simulink model "Lithium-ion"  (R2024b)
settings: Solver=FixedStepAuto  StartTime=0.0  StopTime=10711  FixedStep=0.001  RelTol=1e-3
(part 1 of 3)
settings Model: Creator=holthoff  LastModifiedBy=holthoff

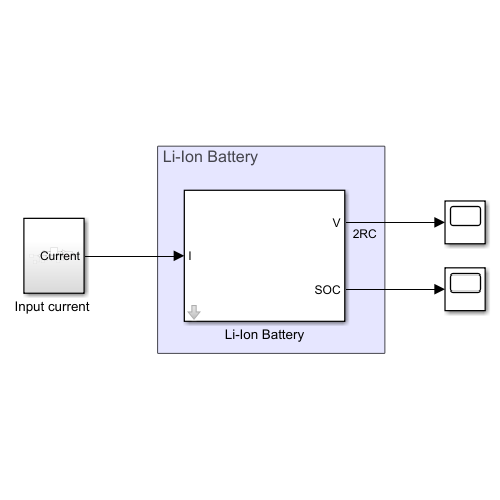
[thumbnail: Simulink's stored preview of the top-level diagram]
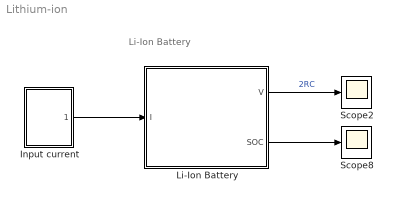
== system Lithium-ion ==
  note: Li-Ion Battery
  "Input current " : Subsystem
  Li-Ion Battery : Subsystem  mask{RCap=3, NomV=5, soc=20, Battime=10}
      mask prompts: RCap "Rated Capacity (Ah)"; NomV "Nominal Voltage (V)"; soc "Initial SOC (%)"; Battime "Battery Response Time (s)"
  Scope2 : Scope
  Scope8 : Scope
  wires:
  "Input current "/1(Current) -> Li-Ion Battery/1(I)
  Li-Ion Battery/1(V) -> Scope2/1  "2RC"
  Li-Ion Battery/2(SOC) -> Scope8/1
